simulink model "PenduloInvertido"  (R2021a)
settings: Solver=VariableStepAuto  StartTime=0.0  StopTime=10.0  RelTol=1e-3
values from neighbouring files (symbols this model uses):
  b = 0.5    [script.m]
  g = 9.81    [script.m]
  J = 8.3e-3    (= 0.0083)    [script.m]
  l = 0.25    [script.m]
  m = 0.1    [script.m]
  M = 2    [script.m]
settings Model: Creator=taffarel55  LastModifiedBy=taffarel55

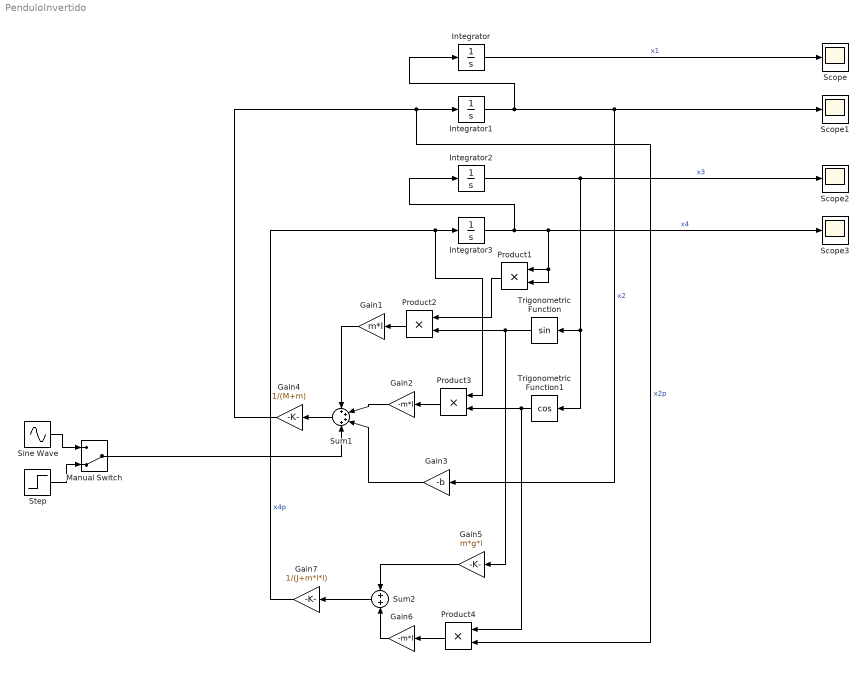
== system PenduloInvertido ==
  Gain1 : Gain  Gain=m*l
  Gain2 : Gain  Gain=-m*l
  Gain3 : Gain  Gain=-b
  Gain4 : Gain  Gain=1/(M+m)
  Gain5 : Gain  Gain=m*g*l
  Gain6 : Gain  Gain=-m*l
  Gain7 : Gain  Gain=1/(J+m*l*l)
  Integrator{,1..3} (4 alike) : Integrator
  Manual Switch : ManualSwitch  CurrentSetting=0
  Product{1..4} (4 alike) : Product
  Scope{,1..3} (4 alike) : Scope
  Sine Wave : Sin  Amplitude=0.1  Frequency=2000*pi  SampleTime=0
  Step : Step  After=0.01  SampleTime=0
  Sum1 : Sum  Inputs=++++
  Sum2 : Sum
  Trigonometric Function : Trigonometry
  Trigonometric Function1 : Trigonometry  Operator=cos
  wires:
  Gain4/1 -> Product4/2, Integrator1/1  "x2p"
  Integrator/1 -> Scope/1  "x1"
  Integrator1/1 -> Integrator/1, Scope1/1, Gain3/1  "x2"
  Integrator3/1 -> Scope3/1, Product1/2, Product1/1, Integrator2/1  "x4"
  Gain7/1 -> Product3/1, Integrator3/1  "x4p"
  Integrator2/1 -> Scope2/1, Trigonometric Function1/1, Trigonometric Function/1  "x3"
  Product1/1 -> Product2/1
  Trigonometric Function/1 -> Gain5/1, Product2/2
  Product2/1 -> Gain1/1
  Trigonometric Function1/1 -> Product4/1, Product3/2
  Product3/1 -> Gain2/1
  Gain3/1 -> Sum1/3
  Gain2/1 -> Sum1/2
  Gain1/1 -> Sum1/1
  Sum1/1 -> Gain4/1
  Gain5/1 -> Sum2/1
  Product4/1 -> Gain6/1
  Gain6/1 -> Sum2/2
  Sum2/1 -> Gain7/1
  Sine Wave/1 -> Manual Switch/1
  Step/1 -> Manual Switch/2
  Manual Switch/1 -> Sum1/4
